simulink model "RRpendulum_digtwin_FSFB_BLDC_noUI"  (R2025b)
settings: Solver=FixedStepAuto  StartTime=0.0  StopTime=inf  FixedStep=0.001  RelTol=1e-3  EnableMultiTasking=on
PreLoadFcn:
  | clear;
  | 
  | if isempty(matlab.project.rootProject)
  |     openProject('C:/Users/u0130154/MATLAB/projects/digtwin_labo/digtwin_labo.prj');
  | end
  | prj = matlab.project.rootProject;
  | 
  | %% Physical parameters
  | load(fullfile(prj.RootFolder, 'data', 'RRpendulum_params_BLDC.mat'), 'params');
  | 
  | %% Controller design (LQR gains)
  | load(fullfile(prj.RootFolder, 'data', 'FSFB_torque_design.mat'), 'design');
  | fsf_par = design.par;
  | 
  | %% UKF observer design
  | load(fullfile(prj.RootFolder, 'data', 'UKF_design.mat'), 'ukf');
  | ukf_par = ukf.par;
  | 
  | %% Swing-up design (Astrom-Furuta energy controller)
  | load(fullfile(prj.RootFolder, 'data', 'swingup_design.mat'), 'swingup');
  | swingup_par = swingup.par;
InitFcn:
  | if isempty(matlab.project.rootProject)
  |     openProject('C:/Users/u0130154/MATLAB/projects/digtwin_labo/digtwin_labo.prj');
  | end
  | prj = matlab.project.rootProject;
  | 
  | %% Physical parameters
  | load(fullfile(prj.RootFolder, 'data', 'RRpendulum_params_BLDC.mat'), 'params');
  | 
  | %% Controller design (LQR gains)
  | load(fullfile(prj.RootFolder, 'data', 'FSFB_torque_design.mat'), 'design');
  | fsf_par = design.par;
  | 
  | %% UKF observer design
  | load(fullfile(prj.RootFolder, 'data', 'UKF_design.mat'), 'ukf');
  | ukf_par = ukf.par;
  | 
  | %% Swing-up design (Astrom-Furuta energy controller)
  | load(fullfile(prj.RootFolder, 'data', 'swingup_design.mat'), 'swingup');
  | swingup_par = swingup.par;
model workspace (MAT data in the model file):
  COUNTS_PER_TURN_MOT = 8192
  COUNTS_PER_TURN_PEND = 2400
  MOTOR_VEL_RESOLUTION_DIV = 4
  PEND_VEL_RESOLUTION_DIV = 1
  T_SAMPLE = 0.001
undefined symbols (not defined in the file): params
libraries: raspberrypiBasiclib x2, simulink x1, digtwin_labo_lib x1
settings Model: SimulationMode=external  ExtModeTrigDuration=2  Creator=u0130154  LastModifiedBy=u0130154
settings SolverCC: PositivePriorityOrder=on  AutoInsertRateTranBlk=on  InsertRTBMode=Always
settings OptimizationCC: EnhancedBackFolding=on  PassReuseOutputArgsAs=Individual arguments  ZeroExternalMemoryAtStartup=off  ZeroInternalMemoryAtStartup=off  MaxStackSize=200000  OptimizeBlockOrder=speed  DifferentSizesBufferReuse=on  OptimizationCustomize=off  EfficientTunableParamExpr=on
settings DebuggingCC: ParameterTunabilityLossMsg=error
settings HardwareCC: ProdBitPerLong=64.0  ProdLargestAtomicInteger=LongLong  ProdLargestAtomicFloat=Double  ProdLongLongMode=on  ProdHWDeviceType=ARM Compatible->ARM Cortex-A (64-bit)
settings RTWCC: SystemTargetFile=ert.tlc  HardwareBoard=Raspberry Pi (64bit)  TLCOptions="-aInlineSetEventsForThisBaseRateFcn=TLC_FALSE -aSuppressMultiTaskScheduler=TLC_FALSE  -aRateBasedStepFcn=0"  TemplateMakefile=ert_default_tmf  Toolchain=GNU GCC Embedded Linux  BuildConfiguration=Faster Runs  Description=Embedded Coder
settings CodeAppCC: ForceParamTrailComments=on  IgnoreCustomStorageClasses=off  OperatorAnnotations=on  SimulinkDataObjDesc=on  SFDataObjDesc=on  InsertBlockDesc=on
settings ERTTargetCC: ExtModeTransport=2.0  ExtModeStaticAlloc=on  ExtModeMexFile=ext_xcp  ExtModeIntrfLevel=Level2 - Open  InlinedParameterPlacement=Hierarchical  CodeReplacementLibrary=ARM Cortex-A CMSIS  SupportVariableSizeSignals=on
settings ExplorerConfigSet: InternalSimMechanicsExplorerSettings=|
  | <ExplorerConfiguration>
  | 
  |   <canonicalview>default</canonicalview>
  | 
  |   <TilePanel>
  |     <TileInfo>
  |       <Tiles Columns="1" Count="1" Height="862" Rows="1" Width="1142">
  |         <Row Weight="1"/>
  |         <Column Weight="1"/>
  |         <Tile Height="1" Width="1" X="0" Y="0"/>
  |       </Tiles>
  |     </TileInfo>
  |     <SceneInfo>
  |       <SceneViewer>
  |         <IsThisViewStd>
  |           <IsStandardView>off</IsStandardView>
  |           <StandardViewName>Front</StandardViewName>
  |         </IsThisViewStd>
  |         <BGColor>
  |           <R>1</R>
  |           <G>1</G>
  |           <B>1</B>
  |           <A>1</A>
  |         </BGColor>
  |         <Camera>
  |           <DoPerspective>off</DoPerspective>
  |           <Position>
  |             <X>-0.7767210645760263</X>
  |             <Y>-0.91604933747716444</Y>
  |             <Z>0.82806995611442047</Z>
  |           </Position>
  |           <Center>
  |             <X>0.16834893542397375</X>
  |             <Y>0.029010662522835545</Y>
  |             <Z>-0.11700004388557958</Z>
  |           </Center>
  |           <Up>
  |             <X>0.40824973039787243</X>
  |             <Y>0.40824973038263623</Y>
  |             <Z>0.81649514099752563</Z>
  |           </Up>
  |           <XLim>0.26600820737762348</XLim>
  |           <YLim>0.26600820737762348</YLim>
  |           <ViewLimDist>0.01</ViewLimDist>
  |         </Camera>
  |       </SceneViewer>
  |     </SceneInfo>
  |   </TilePanel>
  | 
  |   <MechEditorPanel>
  |     <GfxPanelCameraMap/>
  |     <Cameras/>
  |     <VideoCreator>
  |       <IncludeTiles>All</IncludeTiles>
  |       <IncludeTime>on</IncludeTime>
  |       <IncludeWorldFrame>off</IncludeWorldFrame>
  |       <PlaybackSpeedRatio>1</PlaybackSpeedRatio>
  |       <FrameRate>30</FrameRate>
  |       <FrameSize>auto</FrameSize>
  |       <VideoFormat>UncompressedAVI</VideoFormat>
  |     </VideoCreator>
  |   </MechEditorPanel>
  | 
  |   <PlaybackSettings>
  |     <PlaybackSpeedFactor>1</PlaybackSpeedFactor>
  |   </PlaybackSettings>
  | 
  | </ExplorerConfiguration>

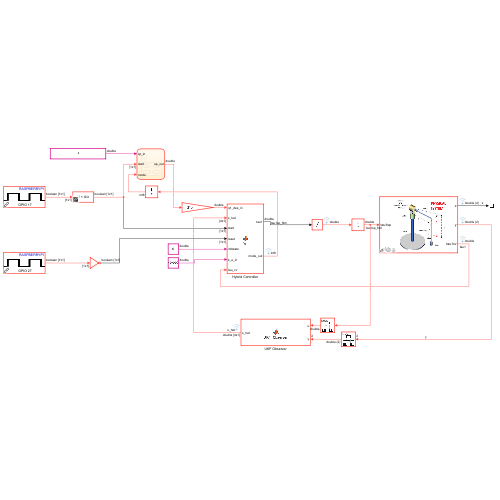
[thumbnail: Simulink's stored preview of the top-level diagram]
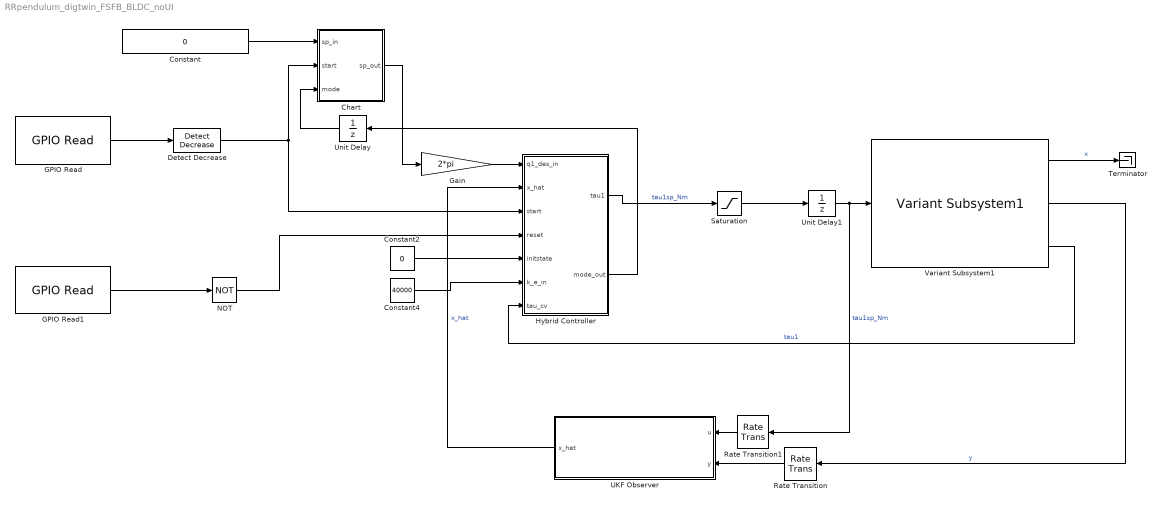
== system RRpendulum_digtwin_FSFB_BLDC_noUI ==
  Chart : Stateflow chart  TreatAsAtomicUnit=on
  Constant : Constant  Value=0
  Constant2 : Constant  Value=0
  Constant4 : Constant  Value=40000
  Detect Decrease : simulink/Logic and Bit Operations/Detect Decrease  vinit=0.0  OutDataTypeStr=boolean
  GPIO Read : raspberrypiBasiclib/GPIO Read  BoardProperty=Pi 4 Model B  gpio=17  SampleTime=-1  blockPlatform=Raspberry Pi  PinNumber=4  board=[]  direction=[]  internalResistor=[]
  GPIO Read1 : raspberrypiBasiclib/GPIO Read  BoardProperty=Pi 4 Model B  gpio=27  SampleTime=-1  blockPlatform=Raspberry Pi  PinNumber=4  board=[]  direction=[]  internalResistor=[]
  Gain : Gain  Gain=2*pi
  Hybrid Controller : MATLAB Function  TreatAsAtomicUnit=on
  NOT : Logic  Operator=NOT  IconShape=distinctive  AllPortsSameDT=off  OutDataTypeStr=boolean
  Rate Transition : RateTransition  OutPortSampleTime=ukf_par.Ts
  Rate Transition1 : RateTransition  OutPortSampleTime=ukf_par.Ts
  Saturation : Saturate  UpperLimit=params.act.u_sat  LowerLimit=-params.act.u_sat
  Terminator : Terminator
  UKF Observer : MATLAB Function  TreatAsAtomicUnit=on
  Unit Delay : UnitDelay  SampleTime=-1  HasFrameUpgradeWarning=on
  Unit Delay1 : UnitDelay  SampleTime=-1  HasFrameUpgradeWarning=on
  Variant Subsystem1 : digtwin_labo_lib/Variant Subsystem1  SystemSampleTime=-1  VariantActivationTime=update diagram  EmptyChoice=off  PassThrough=off  PassThroughVariantControl=(default)  EmptyChoiceVariantControl=(default)  AllowFlexibleInterface=on  Latency=0  AutoFrameSizeCalculation=off
  wires:
  Hybrid Controller/1(tau1) -> Saturation/1  "tau1sp_Nm"
  Variant Subsystem1/3 -> Hybrid Controller/7(tau_cv)  "tau1"
  Variant Subsystem1/1 -> Terminator/1  "x"
  Variant Subsystem1/2 -> Rate Transition/1  "y"
  UKF Observer/1(x_hat) -> Hybrid Controller/2(x_hat)  "x_hat"
  Rate Transition/1 -> UKF Observer/2(y)
  Rate Transition1/1 -> UKF Observer/1(u)
  Constant2/1 -> Hybrid Controller/5(initstate)
  Hybrid Controller/2(mode_out) -> Unit Delay/1
  Constant4/1 -> Hybrid Controller/6(k_e_in)
  Constant/1 -> Chart/1(sp_in)
  Gain/1 -> Hybrid Controller/1(q1_des_in)
  GPIO Read1/1 -> NOT/1
  NOT/1 -> Hybrid Controller/4(reset)
  Detect Decrease/1 -> Hybrid Controller/3(start), Chart/2(start)
  GPIO Read/1 -> Detect Decrease/1
  Chart/1(sp_out) -> Gain/1
  Unit Delay/1 -> Chart/3(mode)
  Saturation/1 -> Unit Delay1/1
  Unit Delay1/1 -> Rate Transition1/1, Variant Subsystem1/1  "tau1sp_Nm"

== matlab function RRpendulum_digtwin_FSFB_BLDC_noUI/Hybrid Controller ==
  data: q1_des_in input; x_hat input; tau1 output; swingup_par parameter; start input; reset input; initstate input; mode_out output; k_e_in input; tau_cv input
function [tau1, mode_out] = fcn(q1_des_in, x_hat, swingup_par, start, reset, initstate, k_e_in, tau_cv)
%#codegen
% Three-phase hybrid controller: swing-up -> stabilize -> FSFB+trajectory


persistent mode q1_ref q1_des dwell_count dropped_count mode_count
if isempty(mode)
    mode = int8(initstate);          % 0=off, 1=stabilize, 2=FSFB+trajectory, 3=swing-up, 4=damping
    q1_ref = 0.0;
    q1_des = 0.0;
    dwell_count = uint32(0);
    dropped_count = uint32(0);
    mode_count = uint32(0);
end

% --- Unpack parameters ---
%k_e = swingup_par.energy.k_e; 
k_e = k_e_in;
alpha_max = swingup_par.energy.alpha_max; 
E0 = swingup_par.energy.E0;
q2_catch = swingup_par.catch.q2_threshold; 
E_catch = swingup_par.catch.E_threshold;
m = swingup_par.plant.m; 
l = swingup_par.plant.l; 
g = swingup_par.plant.g;
r = swingup_par.plant.r; 
Iz_1 = swingup_par.plant.Iz_1;
Kd = swingup_par.fsfb.Kd;  
Nbar = swingup_par.fsfb.Nbar;
max_rate = swingup_par.trajectory.max_rate; 
Ts = swingup_par.fsfb.Ts;
E_latch = swingup_par.catch.E_latch; 
N_dwell = int32(swingup_par.catch.N_dwell);

q1 = x_hat(1); v1 = x_hat(2); q2 = x_hat(3); v2 = x_hat(4);

% --- Wrap q2 into [0, 2*pi), compute signed error from pi ---
q2_err_signed = wrapTo2Pi(q2)-pi;

% --- Pendulum energy (cos is 2pi-periodic, no wrap needed) ---
E = 0.5 * m * l^2 * v2^2 - m * g * l * (cos(q2) + 1);

% --- Catch condition (swing-up -> stabilize) ---
in_catch = (abs(q2_err_signed) < q2_catch) && (abs(E) < E_catch);

if mode == 3 && in_catch
    mode = int8(1);  % enter stabilize phase
end

if reset
    mode = int8(4);  % damping, then turn off
    mode_count = uint32(0);
end

if tau_cv < -0.32 % error reported
    mode = int8(0);  % turn off instantly
    mode_count = uint32(0);
end


if mode == int8(2)
    % === MODE 2: FSFB with q1 trajectory ===
    % Ramp q1_ref
    step = max_rate * Ts;
    err_q1_ref = - q1_ref;
    if err_q1_ref > step
        q1_ref = q1_ref + step;
    elseif err_q1_ref < -step
        q1_ref = q1_ref - step;
    else
        q1_ref = 0;
    end
    % If ref ramped to 0, Ramp q1_des
    if q1_ref == 0
        err_q1 = q1_des_in - q1_des;
        if err_q1 > step
            q1_des = q1_des + step;
        elseif err_q1 < -step
            q1_des = q1_des - step;
        else
            q1_des = q1_des_in;
        end
    else
        q1_des = q1_ref;
    end

    dx = [q1 - q1_ref; v1; q2_err_signed; v2];
    tau1 = Nbar * (q1_des-q1_ref) - Kd * dx;
    
    % Count consecutive samples with not(in_catch)
    if ~in_catch
        dropped_count = dropped_count + uint32(1);
    else
        dropped_count = uint32(0);
    end

    if dropped_count > 500
        mode = int8(0);
        mode_count = uint32(0);
    end

elseif mode == int8(1)
    % === MODE 1: Stabilize (no q1 feedback) ===
    dx_partial = [0; v1; q2_err_signed; v2];
    tau1 = -Kd * dx_partial;

    % Count consecutive samples with |E| < E_latch
    if abs(E) < E_latch
        dwell_count = dwell_count + uint32(1);
    else
        dwell_count = uint32(0);
    end

    % Transition to mode 2 when dwell satisfied
    if dwell_count >= N_dwell
        mode = int8(2);
        mode_count = uint32(0);
        q1_ref = q1;  % latch q1 NOW
    end

    % Count consecutive samples with not(in_catch)
    if ~in_catch
        dropped_count = dropped_count + uint32(1);
    else
        dropped_count = uint32(0);
    end

    if dropped_count > 500
        mode = int8(4);
        mode_count = uint32(0);
    end

elseif mode == int8(3)
    % === MODE 3: Swing-up ===
    E_err = E - E0;
    coupling = v2 * cos(q2);
    if coupling > 0, s = 1.0;
    elseif coupling < 0, s = -1.0;
    else, s = 0.0; end
    alpha1_des = k_e * E_err * s;
    if alpha1_des > alpha_max, alpha1_des = alpha_max;
    elseif alpha1_des < -alpha_max, alpha1_des = -alpha_max; end
    t2 = cos(q1); t3 = sin(q1); t4 = sin(q2);
    Iz1tot = Iz_1 + m*((r*t3 + l*t2*t4)^2 + (r*t2 - l*t3*t4)^2);
    tau1 = Iz1tot * alpha1_des;

elseif mode == int8(4)
    % === MODE 4: damping ===
    tau1 = -x_hat(2)/50;
    if mode_count >= uint32(8000)
        mode = int8(0);
        mode_count = uint32(0);
    else
        mode_count = mode_count + uint32(1);
    end
else
    % === MODE 0: Off ===
    tau1 = 0;
    if start %positive flank on run
        mode = int8(3);
    end

end
mode_out = mode;

== matlab function RRpendulum_digtwin_FSFB_BLDC_noUI/UKF Observer ==
  settings: updateMethod=DISCRETE  sampleTime=ukf_par.Ts
  data: u input size=1; x_hat output size=[4 1]; y input size=[2 1]; ukf_par parameter
function x_hat = UKF_Observer(u, y, ukf_par)
%#codegen
    persistent x_est P_est isInit

    ukf_Q       = ukf_par.noise.Q;
    ukf_R       = ukf_par.noise.R;
    ukf_Wm      = ukf_par.sigma.Wm;
    ukf_Wc      = ukf_par.sigma.Wc;
    ukf_lambda  = ukf_par.sigma.lambda;
    ukf_C       = ukf_par.measurement.C;
    ukf_Ts      = ukf_par.Ts;
    ukf_x0      = ukf_par.ic.x0;
    ukf_P0      = ukf_par.ic.P0;


    if isempty(isInit)
        x_est = zeros(4,1);
        P_est = zeros(4,4);
        x_est(:) = ukf_x0;
        P_est(:) = ukf_P0;
        isInit = true;
    end

    x_new = zeros(4,1);
    P_new = zeros(4,4);
    [x_new, P_new] = ukf_observer_step(x_est, P_est, u, y, ...
        ukf_Q, ukf_R, ukf_Wm, ukf_Wc, ukf_lambda, ukf_C, ukf_Ts);
    x_est = x_new;
    P_est = P_new;

    x_hat = x_est;
end

== stateflow chart RRpendulum_digtwin_FSFB_BLDC_noUI/Chart ==
  state wait
    sp_out = 0;
  state Stabilize
    state stabilized0
      sp_out = sp_in
    state stabilized1
      sp_out = sp_in + 0.25
    state stabilized3
      sp_out = sp_in - 0.25
    state stabilized2
      sp_out = sp_in
    (default) -> stabilized0
    stabilized0 -> stabilized1 : after(0.5,'sec') [start]
    stabilized3 -> stabilized0 : after(0.5,'sec') [start]
    stabilized1 -> stabilized2 : after(0.5,'sec') [start]
    stabilized2 -> stabilized3 : after(0.5,'sec') [start]
  (default) -> wait
  Stabilize -> wait : [mode ~= 2]
  wait -> Stabilize : [mode == 2]
  data: sp_in input; sp_out output; start input; mode input
